simulink library "tqd"  (R2021b)
settings: Solver=VariableStepAuto  StartTime=0.0  StopTime=10.0  RelTol=1e-3
undefined symbols (not defined in the file or in its folder): ATQD_APSDecReq_X_kph, ATQD_APSDecReq_Y_mps2, ATQD_APSDecReqCMD_X_kph, ATQD_APSDecReqTs_X_pct, ATQD_APSDecTimeGain_X_Deg, ATQD_APSDecTimeGain_Y_s, ATQD_APSReqLowSpd_X_Deg, ATQD_AutoHoldReleaseBPS_X_Deg, ATQD_AWDLoadTrqnsGain_X_kg, ATQD_AWDLoadTrqnsGain_Y_pct, ATQD_BOSEnBPSPosn_X_kph, ATQD_BOSMap_X_rpm, ATQD_BOSMap_Y_pct, ATQD_CreepBaseTqD_X_kph, ATQD_CreepBaseTqD_Y_Deg, ATQD_CreepBaseTqR_X_kph, ATQD_CreepBaseTqR_Y_Deg, ATQD_CreepBPSDisPosn_X_Deg, ATQD_CreepBPSDisPosnR_X_Deg, ATQD_CreepBPSEnPosn_X_Deg, ATQD_CreepBPSEnPosnR_X_Deg, ATQD_CreepDeltaTq_X_kph, ATQD_CreepIterm_X_kph, ATQD_CreepIterm_Y_kph, ATQD_CreepItermMaxLimit_X_pct, ATQD_CreepPreloadTime_X_kph, ATQD_CreepPreloadTq_X_kph, ATQD_CreepPreloadTq_Y_s, ATQD_CreepProtTq_X_Deg, ATQD_CreepPterm_X_kph, ATQD_ECOTqMapD_X_rpm, ATQD_ECOTqMapD_Y_pct, ATQD_EOPDTqMapDCon_X_rpm, ATQD_EOPDTqMapDCon_Y_Deg, ATQD_EstInitVehWeight_X_c, ATQD_LHMRollGenMapD_X_rpm, ATQD_LHMRollGenMapD_Y_rpm, ATQD_LHMTqMapD_X_rpm, ATQD_LHMTqMapD_Y_pct, ATQD_NL1TqMapD_X_rpm, ATQD_NL1TqMapD_Y_pct, ATQD_NOPDTqMapDCon_X_rpm, ATQD_NOPDTqMapDCon_Y_Deg, ATQD_NRMRrEDUSpRat_X_rpm, ATQD_NRMRrEDUSpRat_Y_Nm, ATQD_OPDHoldDownRelDelay_X_Deg, ATQD_OPDHoldEnSpd_X_Deg, ATQD_OPDHoldRelDetTime_X_Deg, ATQD_OPDHoldReleaseTq_X_Deg, ATQD_OrigPedTqLowLim_X_Deg, ATQD_OrigPedTqLowLim_Y_pct, ATQD_PedalMapClimbUpLim_X_rpm, ATQD_PedalMapClimbUpLim_Y_Deg, ATQD_PreLoadTq_X_s, ATQD_RollGenMapEL1_X_rpm, ATQD_RollGenMapEL1_Y_rpm, ATQD_SL1TqMapD_X_rpm, ATQD_SL1TqMapD_Y_pct, ATQD_SlideRegenTqGain_X_Gps, ATQD_SlideRegenTqGain_Y_pct ... (+444)
libraries: hcu_lib x70, simulink x61, tqr x1
(part 14 of 14)

== stateflow chart tqd/TQD/TorqueDemand/Signal_convert/Speed Setting Mode/ACC Speed Setting ON/ACCSetSpd_Chart_W ==
  state ACCSetSpeed_W
    (default) -> (junction 431) : {VTQD_ACCSetSpd_kph = ZERO_FLOAT;
        |  VTQD_ACCSavedSetSpd_kph = ZERO_FLOAT;
        |  VTQD_UpDownDetCount_sec = ZERO_FLOAT;
        |  VTQD_StandbyOvrdDetEnd_flg = FALSE;}
    ACCSetSpeed_W -> (junction 538) [order 3]
    (junction 538) -> (junction 552) [order 1] : [VTQD_DistanceUnit_flg == VINP_Distanceunit_flg || VTQD_ACCSavedSetSpd_kph <= ONE_FLOAT]
    (junction 552) -> (junction 431)
    (junction 538) -> (junction 540) [order 2]
    (junction 550) -> (junction 552)
    (junction 431) -> (junction 432) : {VSCP_ActiveDown_flg = FALSE;
        |  VTQD_ActiveUp_flg = FALSE;
        |  VTQD_UpDownTimeCount_sec = ZERO_FLOAT;}
    (junction 540) -> (junction 542) [order 1] : [VINP_Distanceunit_flg == TRUE]
    (junction 540) -> (junction 636) [order 2] : {VTQD_ACCSavedSetSpd_kph = (VTQD_ACCSavedSetSpd_kph * MPH2KPH)}
    (junction 542) -> (junction 599) : {VTQD_ACCSavedSetSpd_kph = (VTQD_ACCSavedSetSpd_kph * KPH2MPH)}
    (junction 432) -> (junction 530) [order 1] : [VINP_ADASACCSta_enum == ENUM_ADASACCSTA_STANDBY ||...
        |  VINP_ADASACCSta_enum == ENUM_ADASACCSTA_OVERRIDE]
    (junction 530) -> (junction 433) [order 1] : [VTQD_SWCSetDownSta_flg == TRUE ||...
        |  VTQD_SWCResUpSta_flg == TRUE]
    (junction 433) -> (junction 419) [order 1] : [VTQD_SWCSetDownSta_flg == TRUE &&...
        |  VTQD_StandbyOvrdDetEnd_flg == FALSE &&...
        |  VTQD_AllowSetSpd_flg == TRUE]
    (junction 432) -> (junction 403) [order 2]
    (junction 530) -> (junction 533) [order 2] : {VTQD_StandbyOvrdDetEnd_flg = FALSE;
        |  VTQD_ACCSetSpd_kph = VTQD_ACCSavedSetSpd_kph;
        |  VTQD_ACCSavedSetSpd_kph = VTQD_ACCSetSpd_kph;
        |  VTQD_DistanceUnit_flg = VINP_Distanceunit_flg;}
    (junction 433) -> (junction 490) [order 2]
    (junction 419) -> (junction 408) : {VTQD_UpDownDetCount_sec = VTQD_UpDownDetCount_sec + task_time_s;}
    (junction 599) -> (junction 602) [order 1] : [VTQD_ACCSavedSetSpd_kph < KTQD_ACCActiveMetSpdLoMPH_mph]
    (junction 636) -> (junction 623) [order 1] : [VTQD_ACCSavedSetSpd_kph < KTQD_ACCActiveMetSpdLo_kph]
    (junction 602) -> (junction 604) : {VTQD_ACCSavedSetSpd_kph = KTQD_ACCActiveMetSpdLoMPH_mph}
    (junction 636) -> (junction 633) [order 2]
    (junction 623) -> (junction 619) : {VTQD_ACCSavedSetSpd_kph = KTQD_ACCActiveMetSpdLo_kph}
    (junction 599) -> (junction 606) [order 2]
    (junction 604) -> (junction 606)
    (junction 619) -> (junction 633)
    (junction 606) -> (junction 613)
    (junction 633) -> (junction 630)
    (junction 630) -> (junction 625) [order 1] : [VTQD_ACCSavedSetSpd_kph > KTQD_ACCActiveMetSpdHi_kph]
    (junction 613) -> (junction 608) [order 1] : [VTQD_ACCSavedSetSpd_kph > KTQD_ACCActiveMetSpdHiMPH_mph]
    (junction 403) -> (junction 395) [order 1] : [(VTQD_SWCSetDownSta_flg == TRUE ||...
        |   VTQD_SWCResUpSta_flg == TRUE) &&...
        |  (VTQD_StandbyOvrdDetEnd_flg == TRUE ||...
        |   VTQD_HoldResDet_flg == TRUE)]
    (junction 490) -> (junction 492) [order 1] : [VINP_ADASACCSta_enum == ENUM_ADASACCSTA_STANDBY &&...
        |  VTQD_SWCResUpSta_flg == TRUE &&...
        |  VTQD_ACCSavedSetSpd_kph > ZERO_FLOAT]
    (junction 408) -> (junction 409) [order 1] : [VTQD_UpDownDetCount_sec > ZERO_FLOAT]
    (junction 409) -> (junction 405) [order 1] : [KTQD_ACCActiveMetSpdHi_raw32 >= VVMC_MeterIndSpeed_raw32 &&...
        |  VVMC_MeterIndSpeed_raw32 >= KTQD_ACCActiveMetSpdLo_raw32]
    (junction 630) -> (junction 632) [order 2]
    (junction 625) -> (junction 628) : {VTQD_ACCSavedSetSpd_kph = KTQD_ACCActiveMetSpdHi_kph}
    (junction 613) -> (junction 615) [order 2]
    (junction 608) -> (junction 612) : {VTQD_ACCSavedSetSpd_kph = KTQD_ACCActiveMetSpdHiMPH_mph}
    (junction 403) -> (junction 396) [order 2] : {VTQD_StandbyOvrdDetEnd_flg = FALSE;
        |  VTQD_HoldResDet_flg = FALSE;}
    (junction 395) -> (junction 399) : {VTQD_StandbyOvrdDetEnd_flg = TRUE;
        |  VTQD_HoldResDet_flg = TRUE;}
    (junction 490) -> (junction 496) [order 2]
    (junction 492) -> (junction 494) : {VTQD_StandbyOvrdDetEnd_flg = TRUE}
    (junction 408) -> (junction 436) [order 2] : {VTQD_ACCSetSpd_kph = VTQD_ACCSavedSetSpd_kph;
        |  VTQD_ACCSavedSetSpd_kph = VTQD_ACCSetSpd_kph;
        |  VTQD_DistanceUnit_flg = VINP_Distanceunit_flg;}
    (junction 409) -> (junction 410) [order 2]
    (junction 405) -> (junction 435) : {VTQD_ACCSetSpd_kph = VVMC_MeterIndSpeed_raw32;
        |  VTQD_ACCSavedSetSpd_kph = VTQD_ACCSetSpd_kph;
        |  VTQD_StandbyOvrdDetEnd_flg = TRUE;
        |  VTQD_UpDownDetCount_sec = ZERO_FLOAT;
        |  VTQD_DistanceUnit_flg = VINP_Distanceunit_flg;}
    (junction 628) -> (junction 632)
    (junction 612) -> (junction 615)
    (junction 632) -> (junction 547)
    (junction 615) -> (junction 544)
    (junction 547) -> (junction 544)
    (junction 544) -> (junction 550)
    (junction 494) -> (junction 496)
    (junction 410) -> (junction 429) [order 1] : [KTQD_ACCActiveMetSpdHi_raw32 < VVMC_MeterIndSpeed_raw32]
    (junction 496) -> (junction 407) : {VTQD_ACCSetSpd_kph = VTQD_ACCSavedSetSpd_kph;
        |  VTQD_ACCSavedSetSpd_kph = VTQD_ACCSetSpd_kph;
        |  VTQD_DistanceUnit_flg = VINP_Distanceunit_flg;}
    (junction 410) -> (junction 420) [order 2] : {VTQD_ACCSetSpd_kph = KTQD_ACCActiveMetSpdLo_raw32;
        |  VTQD_ACCSavedSetSpd_kph = VTQD_ACCSetSpd_kph;
        |  VTQD_StandbyOvrdDetEnd_flg = TRUE;
        |  VTQD_UpDownDetCount_sec = ZERO_FLOAT;
        |  VTQD_DistanceUnit_flg = VINP_Distanceunit_flg;}
    (junction 429) -> (junction 430) : {VTQD_ACCSetSpd_kph = KTQD_ACCActiveMetSpdHi_raw32;
        |  VTQD_ACCSavedSetSpd_kph = VTQD_ACCSetSpd_kph;
        |  VTQD_StandbyOvrdDetEnd_flg = TRUE;
        |  VTQD_UpDownDetCount_sec = ZERO_FLOAT;
        |  VTQD_DistanceUnit_flg = VINP_Distanceunit_flg;}
    (junction 399) -> (junction 396)
    (junction 396) -> (junction 438)
    (junction 438) -> (junction 417) [order 1] : [VINP_ADASACCSta_enum == ENUM_ADASACCSTA_ACTIVE]
    (junction 417) -> (junction 434) [order 1] : [VTQD_SWCSetDownSta_flg == TRUE &&...
        |  VTQD_StandbyOvrdDetEnd_flg == FALSE &&...
        |  VVMC_LVDAACCStatusInformation_flg == FALSE]
    (junction 438) -> (junction 427) [order 2]
    (junction 417) -> (junction 412) [order 2]
    (junction 434) -> (junction 411) : {VTQD_UpDownDetCount_sec = VTQD_UpDownDetCount_sec + task_time_s;}
    (junction 411) -> (junction 437) [order 1] : [VTQD_UpDownDetCount_sec > ZERO_FLOAT]
    (junction 411) -> (junction 406) [order 2] : {VTQD_ACCSetSpd_kph = VTQD_ACCSavedSetSpd_kph;
        |  VTQD_ACCSavedSetSpd_kph = VTQD_ACCSetSpd_kph;
        |  VTQD_DistanceUnit_flg = VINP_Distanceunit_flg;}
    (junction 437) -> (junction 428) : {VTQD_ACCSetSpd_kph = max(KTQD_ACCActiveMetSpdLo_raw32, VTQD_ACCSavedSetSpd_kph - ONE_FLOAT);
        |  VTQD_ACCSavedSetSpd_kph = VTQD_ACCSetSpd_kph;
        |  VSCP_ActiveDown_flg = TRUE;
        |  VTQD_UpDownDetCount_sec = ZERO_FLOAT;
        |  VTQD_UpDownTimeCount_sec = task_time_s;
        |  VTQD_DistanceUnit_flg = VINP_Distanceunit_flg;}
    (junction 427) -> (junction 404) [order 1] : [VINP_ADASACCSta_enum == ENUM_ADASACCSTA_OFF ||...
        |  VINP_ADASACCSta_enum == ENUM_ADASACCSTA_DISABLE||...
        |  VINP_ADASACCSta_enum == ENUM_ADASACCSTA_ERROR]
    (junction 412) -> (junction 510) [order 1] : [VTQD_SWCResUpSta_flg == TRUE]
    (junction 510) -> (junction 413) [order 1] : [VTQD_StandbyOvrdDetEnd_flg == FALSE &&...
        |  VVMC_LVDAACCStatusInformation_flg == FALSE &&...
        |  VTQD_HoldResDet_flg == FALSE]
    (junction 427) -> (junction 422) [order 2] : {VTQD_ACCSetSpd_kph = VTQD_ACCSavedSetSpd_kph;
        |  VTQD_ACCSavedSetSpd_kph = VTQD_ACCSetSpd_kph;
        |  VTQD_DistanceUnit_flg = VINP_Distanceunit_flg;}
    (junction 404) -> (junction 426) : {VTQD_ACCSetSpd_kph = ZERO_FLOAT;
        |  VTQD_ACCSavedSetSpd_kph = VTQD_ACCSetSpd_kph;
        |  VTQD_DistanceUnit_flg = VINP_Distanceunit_flg;}
    (junction 412) -> (junction 522) [order 2]
    (junction 510) -> (junction 512) [order 2]
    (junction 413) -> (junction 414) : {VTQD_UpDownDetCount_sec = VTQD_UpDownDetCount_sec + task_time_s;}
    (junction 512) -> (junction 514) [order 1] : [VTQD_StandbyOvrdDetEnd_flg == FALSE &&...
        |  VVMC_LVDAACCStatusInformation_flg != FALSE]
    (junction 414) -> (junction 415) [order 1] : [VTQD_UpDownDetCount_sec > ZERO_FLOAT]
    (junction 512) -> (junction 519) [order 2]
    (junction 514) -> (junction 516) : {VTQD_HoldResDet_flg = TRUE}
    (junction 414) -> (junction 418) [order 2] : {VTQD_ACCSetSpd_kph = VTQD_ACCSavedSetSpd_kph;
        |  VTQD_ACCSavedSetSpd_kph = VTQD_ACCSetSpd_kph;
        |  VTQD_DistanceUnit_flg = VINP_Distanceunit_flg;}
    (junction 415) -> (junction 421) : {VTQD_ACCSetSpd_kph = min(KTQD_ACCActiveMetSpdHi_raw32, VTQD_ACCSavedSetSpd_kph + ONE_FLOAT);
        |  VTQD_ACCSavedSetSpd_kph = VTQD_ACCSetSpd_kph;
        |  VTQD_ActiveUp_flg = TRUE;
        |  VTQD_UpDownDetCount_sec = ZERO_FLOAT;
        |  VTQD_UpDownTimeCount_sec = task_time_s;
        |  VTQD_DistanceUnit_flg = VINP_Distanceunit_flg;}
    (junction 519) -> (junction 522)
    (junction 516) -> (junction 519)
    (junction 522) -> (junction 416) : {VTQD_ACCSetSpd_kph = VTQD_ACCSavedSetSpd_kph;
        |  VTQD_ACCSavedSetSpd_kph = VTQD_ACCSetSpd_kph;
        |  VTQD_DistanceUnit_flg = VINP_Distanceunit_flg;}
    ACCSetSpeed_W -> (junction 568) [order 1] : [VSCP_ActiveDown_flg == TRUE &&...
        |  VINP_ADASACCSta_enum == ENUM_ADASACCSTA_ACTIVE &&...
        |  VTQD_SWCSetDownSta_flg == TRUE]
    (junction 568) -> (junction 556) [order 1] : [VTQD_DistanceUnit_flg == VINP_Distanceunit_flg]
    (junction 556) -> (junction 423)
    (junction 568) -> (junction 558) [order 2]
    (junction 560) -> (junction 556)
    (junction 423) -> (junction 424) : {VTQD_UpDownTimeCount_sec = VTQD_UpDownTimeCount_sec + task_time_s}
    (junction 558) -> (junction 566) [order 1] : [VINP_Distanceunit_flg == TRUE]
    (junction 558) -> (junction 571) [order 2] : {VTQD_ACCSavedSetSpd_kph = (VTQD_ACCSavedSetSpd_kph * MPH2KPH)}
    (junction 566) -> (junction 557) : {VTQD_ACCSavedSetSpd_kph = (VTQD_ACCSavedSetSpd_kph * KPH2MPH)}
    (junction 424) -> (junction 466) [order 1] : [VTQD_UpDownTimeCount_sec >= KTQD_SetSpdLongPLim_s]
    (junction 424) -> (junction 444) [order 2] : {VTQD_ACCSetSpd_kph = VTQD_ACCSavedSetSpd_kph;
        |  VTQD_ACCSavedSetSpd_kph = VTQD_ACCSetSpd_kph;
        |  VTQD_DistanceUnit_flg = VINP_Distanceunit_flg;}
    (junction 466) -> (junction 478) : {VTQD_ACCSetSpd_kph = max(KTQD_ACCActiveMetSpdLo_raw32, ceil(VTQD_ACCSavedSetSpd_kph / KTQD_SetSpdDeltaLong_kph - ONE_FLOAT) * KTQD_SetSpdDeltaLong_kph);
        |  VTQD_ACCSavedSetSpd_kph = VTQD_ACCSetSpd_kph;
        |  VTQD_UpDownTimeCount_sec = ZERO_FLOAT;
        |  VTQD_DistanceUnit_flg = VINP_Distanceunit_flg;}
    (junction 571) -> (junction 557)
    (junction 557) -> (junction 560)
    ACCSetSpeed_W -> (junction 585) [order 2] : [VTQD_ActiveUp_flg == TRUE &&...
        |  VINP_ADASACCSta_enum == ENUM_ADASACCSTA_ACTIVE &&...
        |  VTQD_SWCResUpSta_flg == TRUE]
    (junction 585) -> (junction 583) [order 1] : [VTQD_DistanceUnit_flg == VINP_Distanceunit_flg]
    (junction 583) -> (junction 479)
    (junction 585) -> (junction 584) [order 2]
    (junction 580) -> (junction 583)
    (junction 479) -> (junction 480) : {VTQD_UpDownTimeCount_sec = VTQD_UpDownTimeCount_sec + task_time_s}
    (junction 584) -> (junction 576) [order 1] : [VINP_Distanceunit_flg == TRUE]
    (junction 584) -> (junction 573) [order 2] : {VTQD_ACCSavedSetSpd_kph = (VTQD_ACCSavedSetSpd_kph * MPH2KPH)}
    (junction 576) -> (junction 582) : {VTQD_ACCSavedSetSpd_kph = (VTQD_ACCSavedSetSpd_kph * KPH2MPH)}
    (junction 480) -> (junction 463) [order 1] : [VTQD_UpDownTimeCount_sec >= KTQD_SetSpdLongPLim_s]
    (junction 480) -> (junction 455) [order 2] : {VTQD_ACCSetSpd_kph = VTQD_ACCSavedSetSpd_kph;
        |  VTQD_ACCSavedSetSpd_kph = VTQD_ACCSetSpd_kph;
        |  VTQD_DistanceUnit_flg = VINP_Distanceunit_flg;}
    (junction 463) -> (junction 461) : {VTQD_ACCSetSpd_kph = min(KTQD_ACCActiveMetSpdHi_raw32, floor(VTQD_ACCSavedSetSpd_kph / KTQD_SetSpdDeltaLong_kph + ONE_FLOAT) * KTQD_SetSpdDeltaLong_kph);
        |  VTQD_ACCSavedSetSpd_kph = VTQD_ACCSetSpd_kph;
        |  VTQD_UpDownTimeCount_sec = ZERO_FLOAT;
        |  VTQD_DistanceUnit_flg = VINP_Distanceunit_flg;}
    (junction 573) -> (junction 582)
    (junction 582) -> (junction 580)
  data: VINP_ADASACCSta_enum input uint8; VTQD_SWCResUpSta_flg input boolean; VTQD_SWCSetDownSta_flg input boolean; VVMC_MeterIndSpeed_raw32 input single; KTQD_ACCActiveMetSpdHi_raw32 input uint8; VINP_Distanceunit_flg input boolean; KTQD_ACCActiveMetSpdLo_raw32 input uint8; VTQD_ACCSetSpd_kph output single; KTQD_SetSpdDeltaLong_kph input uint8; VTQD_ACCSavedSetSpd_kph local single; ENUM_ADASACCSTA_STANDBY parameter uint8; ZERO_FLOAT parameter single; TRUE parameter boolean; ENUM_ADASACCSTA_ACTIVE parameter uint8; ONE_FLOAT parameter single; FALSE parameter boolean; VSCP_ActiveDown_flg local boolean; VTQD_UpDownTimeCount_sec local single; VTQD_ActiveUp_flg local boolean; KTQD_SetSpdLongPLim_s input single; VTQD_UpDownDetCount_sec local single; ENUM_ADASACCSTA_OVERRIDE parameter uint8; VTQD_StandbyOvrdDetEnd_flg local boolean; ENUM_ADASACCSTA_DISABLE parameter; ENUM_ADASACCSTA_OFF parameter; ENUM_ADASACCSTA_ERROR parameter; VVMC_LVDAACCStatusInformation_flg input; VTQD_HoldResDet_flg local boolean; VTQD_AllowSetSpd_flg input; task_time_s input; VTQD_DistanceUnit_flg local boolean; KPH2MPH parameter; MPH2KPH parameter; KTQD_ACCActiveMetSpdLo_kph parameter; KTQD_ACCActiveMetSpdLoMPH_mph parameter; KTQD_ACCActiveMetSpdHiMPH_mph parameter; KTQD_ACCActiveMetSpdHi_kph parameter
